simulink model "pid_tune"  (R2022a)
settings: Solver=FixedStepAuto  StartTime=0.0  StopTime=42.0  RelTol=1e-3
libraries: mbedblockslib x6, slpidlib x2, slctrlblks x2, hdlsllib x1
settings Model: PacingRate=2  ExtModeTrigDuration=10  Creator=MATLAB  LastModifiedBy=FUGAZI
settings SolverCC: AutoInsertRateTranBlk=on
settings OptimizationCC: EnhancedBackFolding=on  PassReuseOutputArgsAs=Individual arguments  ZeroExternalMemoryAtStartup=off  ZeroInternalMemoryAtStartup=off  MaxStackSize=64  OptimizeBlockOrder=speed  DifferentSizesBufferReuse=on  OptimizationCustomize=off  EfficientTunableParamExpr=on
settings DebuggingCC: ParameterTunabilityLossMsg=error
settings HardwareCC: ProdBitPerPointer=32  ProdBitPerSizeT=32  ProdBitPerPtrDiffT=32  ProdLargestAtomicInteger=Long  ProdLargestAtomicFloat=Double  ProdWordSize=32  ProdLongLongMode=on  ProdHWDeviceType=ARM Compatible->ARM Cortex
settings SFSimCC: MATLABDynamicMemAlloc=off
settings RTWCC: SystemTargetFile=ert.tlc  HardwareBoard=STM32 Nucleo L476RG  TemplateMakefile=ert_default_tmf  Toolchain=GNU Tools for ARM Embedded Processors
settings CodeAppCC: ForceParamTrailComments=on  IgnoreCustomStorageClasses=off  OperatorAnnotations=on  SimulinkDataObjDesc=on  SFDataObjDesc=on  InsertBlockDesc=on
settings ERTTargetCC: ExtModeTransport=3  ExtModeStaticAlloc=on  ExtModeStaticAllocSize=2000  ExtModeMexFile=ext_xcp  ExtModeIntrfLevel=Level2 - Open

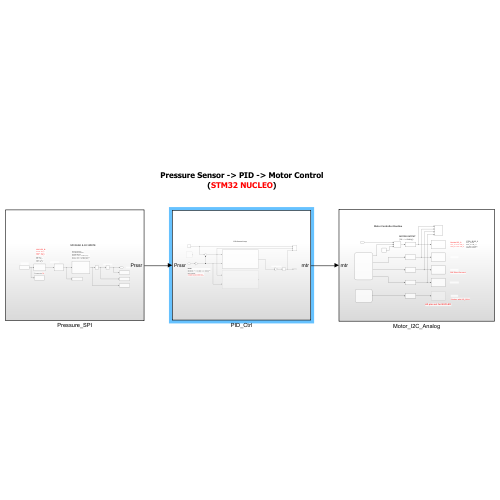
[thumbnail: Simulink's stored preview of the top-level diagram]
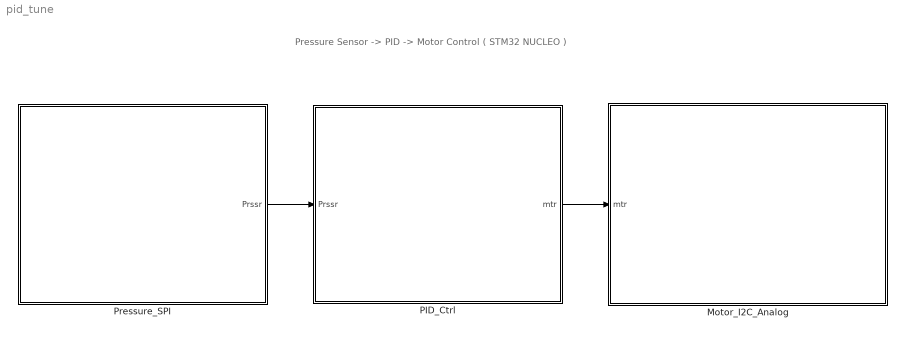
== system pid_tune ==
  note: Pressure Sensor -> PID -> Motor Control
      | ( STM32 NUCLEO )
  Motor_I2C_Analog : Subsystem
  PID_Ctrl : Subsystem
  Pressure_SPI : Subsystem
  wires:
  PID_Ctrl/1(mtr) -> Motor_I2C_Analog/1(mtr)
  Pressure_SPI/1(Prssr) -> PID_Ctrl/1(Prssr)

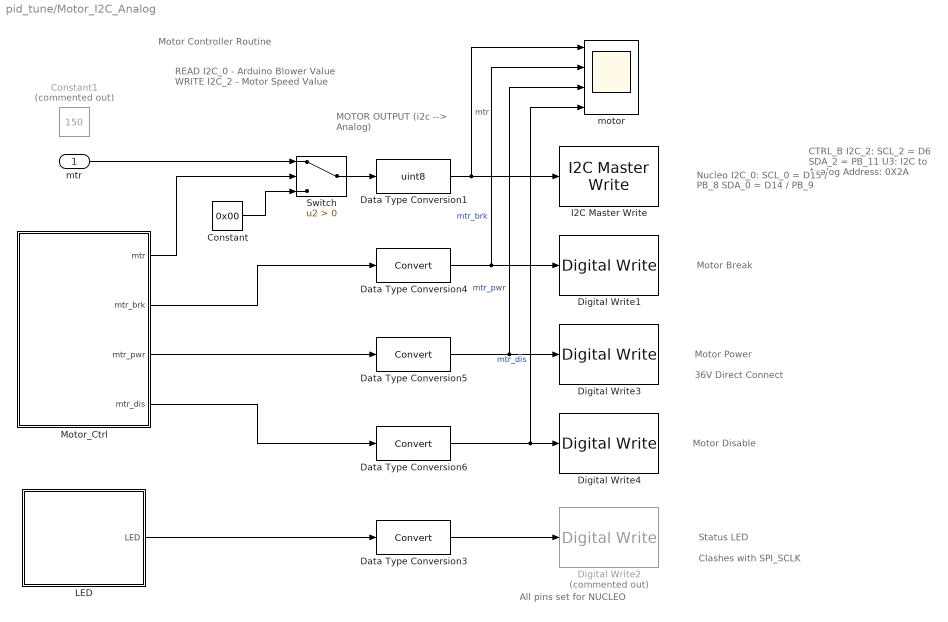
== system pid_tune/Motor_I2C_Analog ==
  note: All pins set for NUCLEO
  note: Motor Controller Routine
  note: Status LED
  note: READ  I2C_0  - Arduino Blower Value
      | WRITE I2C_2 - Motor Speed Value
  note: Motor Power
  note: MOTOR OUTPUT
      | (i2c --> Analog)
  note: Motor Break
  note: Motor Disable
  note: CTRL_B I2C_2:
      | SCL_2 = D6
      | SDA_2 = PB_11
      | U3: I2C to Analog
      | Address: 0X2A
  note: 36V Direct Connect
  note: Nucleo I2C_0:
      | SCL_0 = D15 / PB_8
      | SDA_0 = D14 / PB_9
  note: Clashes with SPI_SCLK
  mtr : Inport
  Constant : Constant  Value=0x00
  Constant1 : Constant  Commented=on  Value=150
  Data Type Conversion1 : DataTypeConversion  OutDataTypeStr=uint8  SaturateOnIntegerOverflow=off  RndMeth=Floor
  Data Type Conversion{3..6} (4 alike) : DataTypeConversion  SaturateOnIntegerOverflow=off  RndMeth=Floor
  Digital Write1 : mbedblockslib/Digital Write  Pin=PA_8  Direction=output
      settings: SourceProductBaseCode=MICROBIT,NUCLEO,STMICRODIS
  Digital Write2 : mbedblockslib/Digital Write  Commented=on  Pin=PA_5  Direction=output
      settings: SourceProductBaseCode=MICROBIT,NUCLEO,STMICRODIS
  Digital Write3 : mbedblockslib/Digital Write  Pin=PB_4  Direction=output
      settings: SourceProductBaseCode=MICROBIT,NUCLEO,STMICRODIS
  Digital Write4 : mbedblockslib/Digital Write  Pin=PB_10  Direction=output
      settings: SourceProductBaseCode=MICROBIT,NUCLEO,STMICRODIS
  I2C Master Write : mbedblockslib/I2C Master Write  I2CModule=0  Mode=Master  SlaveAddress=uint8(hex2dec('2A'))  SlaveByteOrder=BigEndian  Direction=Transmitter  RegisterAddressMode=on  RegisterAddress=uint8(hex2dec('10'))  SlaveDataType=uint8  DataLength=2  NoAck=off  RepeatedStart=off  OutputStatus=off
      settings: SourceProductBaseCode=MICROBIT,NUCLEO,STMICRODIS
  LED : Stateflow chart  TreatAsAtomicUnit=on
  Motor_Ctrl : Stateflow chart  TreatAsAtomicUnit=on
  Switch : Switch  Criteria=u2 > Threshold  SaturateOnIntegerOverflow=off  InputSameDT=off
  motor : Scope  NumInputPorts=4
  wires:
  Data Type Conversion5/1 -> Digital Write3/1, motor/3  "mtr_pwr"
  Switch/1 -> Data Type Conversion1/1
  Motor_Ctrl/1(mtr) -> Switch/2
  Motor_Ctrl/3(mtr_pwr) -> Data Type Conversion5/1
  Data Type Conversion6/1 -> motor/4, Digital Write4/1  "mtr_dis"
  Motor_Ctrl/2(mtr_brk) -> Data Type Conversion4/1
  Data Type Conversion3/1 -> Digital Write2/1
  Motor_Ctrl/4(mtr_dis) -> Data Type Conversion6/1
  Data Type Conversion4/1 -> Digital Write1/1, motor/2  "mtr_brk"
  Data Type Conversion1/1 -> motor/1, I2C Master Write/1  "mtr"
  LED/1(LED) -> Data Type Conversion3/1
  Constant/1 -> Switch/3
  mtr/1 -> Switch/1

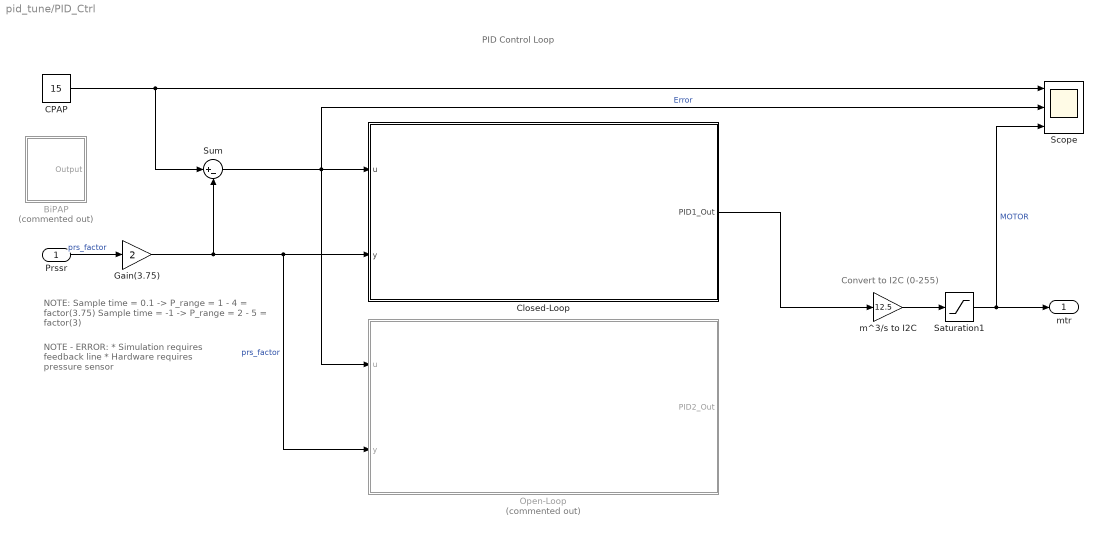
== system pid_tune/PID_Ctrl ==
  note: NOTE:
      | Sample time = 0.1 -> P_range = 1 - 4 = factor(3.75)
      | Sample time = -1 -> P_range = 2 - 5 = factor(3)
  note: PID Control Loop
  note: Convert to I2C (0-255)
  note: NOTE - ERROR:
      | * Simulation requires feedback line
      | * Hardware requires pressure sensor
  Prssr : Inport
  BiPAP : Stateflow chart  Commented=on  TreatAsAtomicUnit=on
  CPAP : Constant  Value=15
  Closed-Loop : Subsystem
  Gain(3.75) : Gain  Gain=2
  Open-Loop : Subsystem  Commented=on
  Saturation1 : Saturate  UpperLimit=180  LowerLimit=0
  Scope : Scope  NumInputPorts=3
  Sum : Sum  Inputs=|+-
  m^3/s to I2C : Gain  Gain=12.5
  mtr : Outport
  wires:
  Saturation1/1 -> Scope/3, mtr/1  "MOTOR"
  m^3/s to I2C/1 -> Saturation1/1
  Prssr/1 -> Gain(3.75)/1  "prs_factor"
  Sum/1 -> Scope/2, Open-Loop/1(u), Closed-Loop/1(u)  "Error"
  Closed-Loop/1(PID1_Out) -> m^3/s to I2C/1
  CPAP/1 -> Sum/1, Scope/1
  Gain(3.75)/1 -> Open-Loop/2(y), Closed-Loop/2(y), Sum/2  "prs_factor"

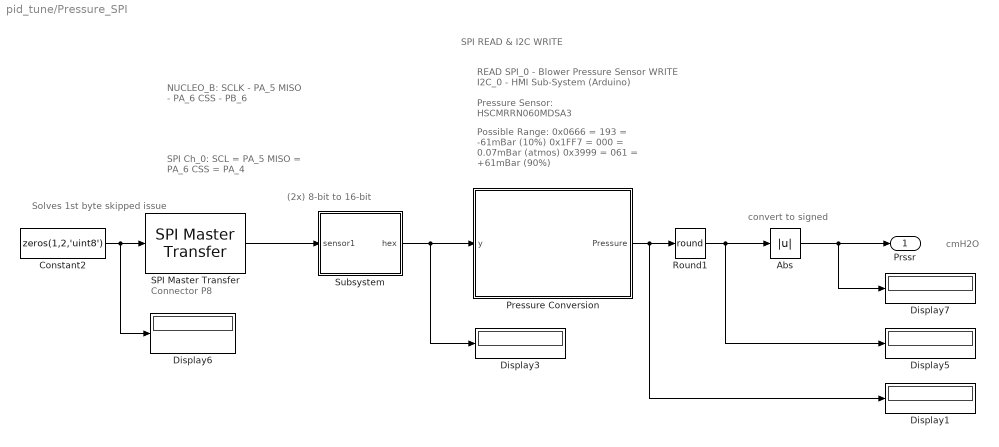
== system pid_tune/Pressure_SPI ==
  note: Pressure Sensor:
      | HSCMRRN060MDSA3
  note: Connector P8
  note: cmH2O
  note: convert to signed
  note: (2x) 8-bit to 16-bit
  note: SPI READ & I2C WRITE
  note: READ SPI_0  -  Blower Pressure Sensor
      | WRITE I2C_0 - HMI Sub-System (Arduino)
  note: SPI Ch_0:
      | SCL = PA_5
      | MISO = PA_6
      | CSS = PA_4
  note: Solves 1st byte
      | skipped issue
  note: Possible Range:
      | 0x0666 = 193 = -61mBar (10%)
      | 0x1FF7 = 000 = 0.07mBar (atmos)
      | 0x3999 = 061 = +61mBar (90%)
  note: NUCLEO_B:
      | SCLK - PA_5
      | MISO - PA_6
      | CSS - PB_6
  Abs : Abs  SaturateOnIntegerOverflow=off
  Constant2 : Constant  Value=zeros(1,2,'uint8')  OutDataTypeStr=uint8  SampleTime=0.1
  Display{1,3,5..7} (5 alike) : Display
      Display3 settings: Format=hex (Stored Integer)
      Display6 settings: Format=hex (Stored Integer)
  Pressure Conversion : Subsystem
  Round1 : Rounding  Operator=round
  SPI Master Transfer : mbedblockslib/SPI Master Transfer  SPIModule=0  Mode=Master  BusSpeed=uint32( 1000000 )  Pin=PB_6  FirstBitToTransfer=Most significant bit (MSB)  ClockMode=0  BlockFunction=Transfer  RegisterAddress=0  OutputDataType=int8  OutputDataLength=1  UseCustomSSPin=Explicit GPIO calls  ActiveLowSSPin=Active low
      settings: SourceProductBaseCode=MICROBIT,NUCLEO,STMICRODIS
  Subsystem : Subsystem
  Prssr : Outport
  wires:
  SPI Master Transfer/1 -> Subsystem/1(sensor1)
  Subsystem/1(hex) -> Pressure Conversion/1(y), Display3/1
  Constant2/1 -> SPI Master Transfer/1, Display6/1
  Round1/1 -> Abs/1, Display5/1
  Pressure Conversion/1(Pressure) -> Display1/1, Round1/1
  Abs/1 -> Display7/1, Prssr/1

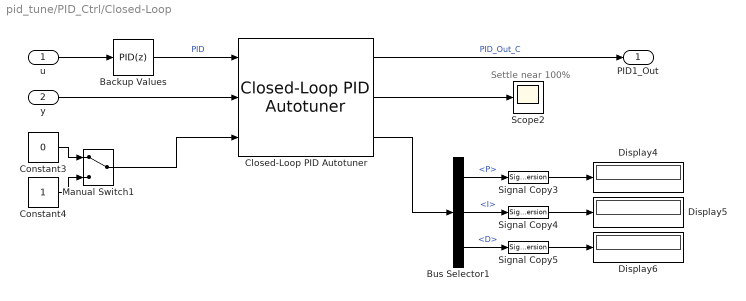
== system pid_tune/PID_Ctrl/Closed-Loop ==
  note: Settle near 100%
  u : Inport
  y : Inport  Port=2
  Backup Values : slpidlib/PID Controller  Controller=PID  Form=Parallel  TimeDomain=Discrete-time  UseExternalTs=off  SampleTime=-1  IntegratorMethod=Forward Euler  FilterMethod=Forward Euler  ControllerParametersSource=internal  P=5  I=25  UseKiTs=off  D=1  N=80  UseFilter=on  TunerSelectOption=Transfer Function Based (PID Tuner App)  InitialConditionSource=internal  InitialConditionForIntegrator=0  InitialConditionForFilter=0  DifferentiatorICPrevScaledInput=0  ExternalReset=none  TrackingMode=off  Kt=1  LimitOutput=off  SatLimitsSource=internal  UpperSaturationLimit=1  LowerSaturationLimit=0  LinearizeAsGain=off  AntiWindupMode=none  Kb=1  POutMin=[]  POutMax=[]  IOutMin=[]  IOutMax=[]  DOutMin=[]  DOutMax=[]  NOutMin=[]  NOutMax=[]  SumOutMin=[]  SumOutMax=[]  SaturationOutMin=[]  SaturationOutMax=[]  PParamMin=[]  PParamMax=[]  IParamMin=[]  IParamMax=[]  DParamMin=[]  DParamMax=[]  NParamMin=[]  NParamMax=[]  KbParamMin=[]  KbParamMax=[]  KtParamMin=[]  KtParamMax=[]  KbOutMin=[]  KbOutMax=[]  KtOutMin=[]  KtOutMax=[]  IntegratorOutMin=[]  IntegratorOutMax=[]  FilterOutMin=[]  FilterOutMax=[]  SumI1OutMin=[]  SumI1OutMax=[]  SumI2OutMin=[]  SumI2OutMax=[]  SumI3OutMin=[]  SumI3OutMax=[]  SumI4OutMin=[]  SumI4OutMax=[]  SumDOutMin=[]  SumDOutMax=[]  DifferentiatorOutMin=[]  DifferentiatorOutMax=[]  FilterDiffOutCoefMin=[]  FilterDiffOutCoefMax=[]  ReciprocalOutMin=[]  ReciprocalOutMax=[]  SumDenOutMin=[]  SumDenOutMax=[]  SumNumOutMin=[]  SumNumOutMax=[]  DivideOutMin=[]  DivideOutMax=[]  UdiffTsProdOutMin=[]  UdiffTsProdOutMax=[]  NTsProdOutMin=[]  NTsProdOutMax=[]  UintegralTsProdOutMin=[]  UintegralTsProdOutMax=[]  UngainTsProdOutMin=[]  UngainTsProdOutMax=[]  IntegratorContinuousStateAttributes=''  IntegratorStateMustResolveToSignalObject=off  IntegratorRTWStateStorageClass=Auto  FilterContinuousStateAttributes=''  FilterStateMustResolveToSignalObject=off  FilterRTWStateStorageClass=Auto  ParallelPVariant=InternalParameters  IdealPVariant=Disabled  IVariant=InternalParameters  DVariant=InternalParameters  IntegratorVariant=Discrete  SatVariant=Disabled  AWVariant=Passthrough  PCopyVariant=Disabled  TRVariant=Disabled  FdbkBlocksVariant=Forward  IdealPFdbkVariant=Disabled  SatFdbkVariant=Disabled  DerivativeFilterVariant=ForwardEulerFilter  NVariant=InternalParameters  NCopyVariant=Disabled  FilterICVariant=InternalICsFilter  IntegratorICVariant=InternalICs  ExternalResetVariant=Disabled  TRSumVariant=Passthrough  SumFdbkVariant=Disabled  SumVariant=Sum_PID  TsampFilterVariant=InternalTs  TsampNgainVariant=Passthrough  TsampIntegralVariant=Passthrough  ExternalSaturationOutDataTypeStr=Inherit: Same as second input  aMode=0
  Bus Selector1 : BusSelector  OutputSignals=P,I,D
  Closed-Loop PID Autotuner : slctrlblks/Closed-Loop PID Autotuner  PIDType=PID  PIDForm=Parallel  TimeDomain=discrete-time  DiscreteTs=-1  TuningTs=0.2  UseTuningTs=off  IntegratorFormula=Forward Euler  FilterFormula=Forward Euler  ContinuousTs=0.02  Bandwidth=28  UseExternalWC=off  TargetPM=45  UseExternalPM=off  UseExternalAchievedPM=off  ExperimentMode=Superposition  PlantType=Stable  PlantSign=Positive  AmpSine=10  UseExternalAmpSine=off  UseExternalFRD=off  UseExternalU0=off  UseCompanion=off  NotDeployTuningModule=off  UsePLCCoder=off  OutputMode=control action + perturbation  BlockDataType=double  UseConnectedPID=on  blockpath=[]  tunedP=0  tunedI=0  tunedD=0  tunedN=100  tunedPM=0  EstimationWindowSize=3  UseExternalTuningParams=off  OutputChoice=VariantCandD  SingleMultiRateVariant=SingleSamplingRate  ExperimentModeVariant=VariantSuperimposed  NumEstimationPeriods=4  NumSettlingPeriods=2
      settings: SourceProductBaseCode=SD
  Constant3 : Constant  Value=0
  Constant4 : Constant
  Display4 : Display
  Display5 : Display
  Display6 : Display
  Manual Switch1 : ManualSwitch
  Scope2 : Scope
  Signal Copy3 : SignalConversion  OverrideOpt=off
  Signal Copy4 : SignalConversion  OverrideOpt=off
  Signal Copy5 : SignalConversion  OverrideOpt=off
  PID1_Out : Outport
  wires:
  Signal Copy4/1 -> Display5/1
  Bus Selector1/3 -> Signal Copy5/1  "<D>"
  Closed-Loop PID Autotuner/1 -> PID1_Out/1  "PID_Out_C"
  Constant4/1 -> Manual Switch1/2
  Constant3/1 -> Manual Switch1/1
  Bus Selector1/2 -> Signal Copy4/1  "<I>"
  Signal Copy3/1 -> Display4/1
  Bus Selector1/1 -> Signal Copy3/1  "<P>"
  u/1 -> Backup Values/1
  Signal Copy5/1 -> Display6/1
  Backup Values/1 -> Closed-Loop PID Autotuner/1  "PID"
  Closed-Loop PID Autotuner/3 -> Bus Selector1/1
  Closed-Loop PID Autotuner/2 -> Scope2/1
  y/1 -> Closed-Loop PID Autotuner/2
  Manual Switch1/1 -> Closed-Loop PID Autotuner/3

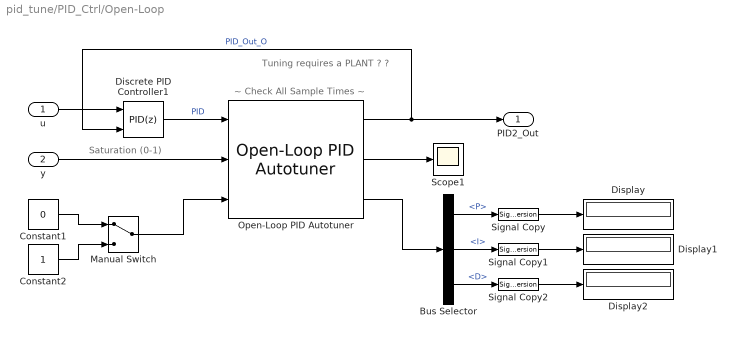
== system pid_tune/PID_Ctrl/Open-Loop ==
  note: Tuning requires
      | a PLANT ? ?
  note: ~ Check All Sample Times ~
  note: Saturation (0-1)
  u : Inport
  y : Inport  Port=2
  Bus Selector : BusSelector  OutputSignals=P,I,D
  Constant1 : Constant  Value=0
  Constant2 : Constant
  Discrete PID Controller1 : slpidlib/PID Controller  Controller=PID  Form=Parallel  TimeDomain=Discrete-time  UseExternalTs=off  SampleTime=-1  IntegratorMethod=Forward Euler  FilterMethod=Forward Euler  ControllerParametersSource=internal  P=90  I=140  UseKiTs=off  D=4  N=100  UseFilter=on  TunerSelectOption=Transfer Function Based (PID Tuner App)  InitialConditionSource=internal  InitialConditionForIntegrator=0  InitialConditionForFilter=0  DifferentiatorICPrevScaledInput=0  ExternalReset=none  TrackingMode=on  Kt=1  LimitOutput=off  SatLimitsSource=internal  UpperSaturationLimit=1  LowerSaturationLimit=0  LinearizeAsGain=off  AntiWindupMode=none  Kb=1  POutMin=[]  POutMax=[]  IOutMin=[]  IOutMax=[]  DOutMin=[]  DOutMax=[]  NOutMin=[]  NOutMax=[]  SumOutMin=[]  SumOutMax=[]  SaturationOutMin=[]  SaturationOutMax=[]  PParamMin=[]  PParamMax=[]  IParamMin=[]  IParamMax=[]  DParamMin=[]  DParamMax=[]  NParamMin=[]  NParamMax=[]  KbParamMin=[]  KbParamMax=[]  KtParamMin=[]  KtParamMax=[]  KbOutMin=[]  KbOutMax=[]  KtOutMin=[]  KtOutMax=[]  IntegratorOutMin=[]  IntegratorOutMax=[]  FilterOutMin=[]  FilterOutMax=[]  SumI1OutMin=[]  SumI1OutMax=[]  SumI2OutMin=[]  SumI2OutMax=[]  SumI3OutMin=[]  SumI3OutMax=[]  SumI4OutMin=[]  SumI4OutMax=[]  SumDOutMin=[]  SumDOutMax=[]  DifferentiatorOutMin=[]  DifferentiatorOutMax=[]  FilterDiffOutCoefMin=[]  FilterDiffOutCoefMax=[]  ReciprocalOutMin=[]  ReciprocalOutMax=[]  SumDenOutMin=[]  SumDenOutMax=[]  SumNumOutMin=[]  SumNumOutMax=[]  DivideOutMin=[]  DivideOutMax=[]  UdiffTsProdOutMin=[]  UdiffTsProdOutMax=[]  NTsProdOutMin=[]  NTsProdOutMax=[]  UintegralTsProdOutMin=[]  UintegralTsProdOutMax=[]  UngainTsProdOutMin=[]  UngainTsProdOutMax=[]  IntegratorContinuousStateAttributes=''  IntegratorStateMustResolveToSignalObject=off  IntegratorRTWStateStorageClass=Auto  FilterContinuousStateAttributes=''  FilterStateMustResolveToSignalObject=off  FilterRTWStateStorageClass=Auto  ParallelPVariant=InternalParameters  IdealPVariant=Disabled  IVariant=InternalParameters  DVariant=InternalParameters  IntegratorVariant=Discrete  SatVariant=Disabled  AWVariant=Passthrough  PCopyVariant=Disabled  TRVariant=Enabled  FdbkBlocksVariant=Forward  IdealPFdbkVariant=Disabled  SatFdbkVariant=Disabled  DerivativeFilterVariant=ForwardEulerFilter  NVariant=InternalParameters  NCopyVariant=Disabled  FilterICVariant=InternalICsFilter  IntegratorICVariant=InternalICs  ExternalResetVariant=Disabled  TRSumVariant=TrackingMode  SumFdbkVariant=Disabled  SumVariant=Sum_PID  TsampFilterVariant=InternalTs  TsampNgainVariant=Passthrough  TsampIntegralVariant=Passthrough  ExternalSaturationOutDataTypeStr=Inherit: Same as second input  aMode=0
  Display : Display
  Display1 : Display
  Display2 : Display
  Manual Switch : ManualSwitch
  Open-Loop PID Autotuner : slctrlblks/Open-Loop PID Autotuner  PIDType=PI  PIDForm=Parallel  TimeDomain=discrete-time  DiscreteTs=0.1  IntegratorFormula=Forward Euler  FilterFormula=Forward Euler  ContinuousTs=0.02  Bandwidth=1  UseExternalWC=off  TargetPM=60  UseExternalPM=off  UseExternalAchievedPM=off  AmpSine=1  UseExternalAmpSine=off  EstimateDCGain=on  AmpStep=1  UseExternalAmpStep=off  UseExternalFRD=off  UseExternalU0=off  UseExternalDCGain=off  NotDeployTuningModule=off  UsePLCCoder=off  BlockDataType=double  UseConnectedPID=on  blockpath=[]  tunedP=0  tunedI=0  tunedD=0  tunedN=100  tunedPM=0  EstimationWindowSize=3
      settings: SourceProductBaseCode=SD
  Scope1 : Scope
  Signal Copy : SignalConversion  OverrideOpt=off
  Signal Copy1 : SignalConversion  OverrideOpt=off
  Signal Copy2 : SignalConversion  OverrideOpt=off
  PID2_Out : Outport
  wires:
  Bus Selector/2 -> Signal Copy1/1  "<I>"
  Bus Selector/1 -> Signal Copy/1  "<P>"
  Constant2/1 -> Manual Switch/2
  Signal Copy/1 -> Display/1
  Open-Loop PID Autotuner/1 -> Discrete PID Controller1/2, PID2_Out/1  "PID_Out_O"
  Signal Copy2/1 -> Display2/1
  Constant1/1 -> Manual Switch/1
  Bus Selector/3 -> Signal Copy2/1  "<D>"
  Signal Copy1/1 -> Display1/1
  Open-Loop PID Autotuner/2 -> Scope1/1
  Discrete PID Controller1/1 -> Open-Loop PID Autotuner/1  "PID"
  Manual Switch/1 -> Open-Loop PID Autotuner/3
  Open-Loop PID Autotuner/3 -> Bus Selector/1
  y/1 -> Open-Loop PID Autotuner/2
  u/1 -> Discrete PID Controller1/1

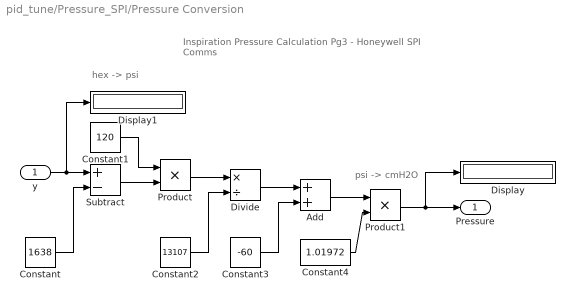
== system pid_tune/Pressure_SPI/Pressure Conversion ==
  note: psi -> cmH2O
  note: Inspiration Pressure Calculation
      | Pg3 - Honeywell SPI Comms
  note: hex -> psi
  y : Inport
  Add : Sum
  Constant : Constant  Value=1638
  Constant1 : Constant  Value=120
  Constant2 : Constant  Value=13107
  Constant3 : Constant  Value=-60
  Constant4 : Constant  Value=1.01972
  Display : Display
  Display1 : Display
      settings: Format=hex (Stored Integer)
  Divide : Product  Inputs=*/
  Product : Product
  Product1 : Product
  Subtract : Sum  Inputs=+-
  Pressure : Outport
  wires:
  Constant/1 -> Subtract/2
  Subtract/1 -> Product/2
  Constant1/1 -> Product/1
  Product/1 -> Divide/1
  Constant2/1 -> Divide/2
  Constant3/1 -> Add/2
  Divide/1 -> Add/1
  Add/1 -> Product1/1
  Constant4/1 -> Product1/2
  Product1/1 -> Pressure/1, Display/1
  y/1 -> Display1/1, Subtract/1

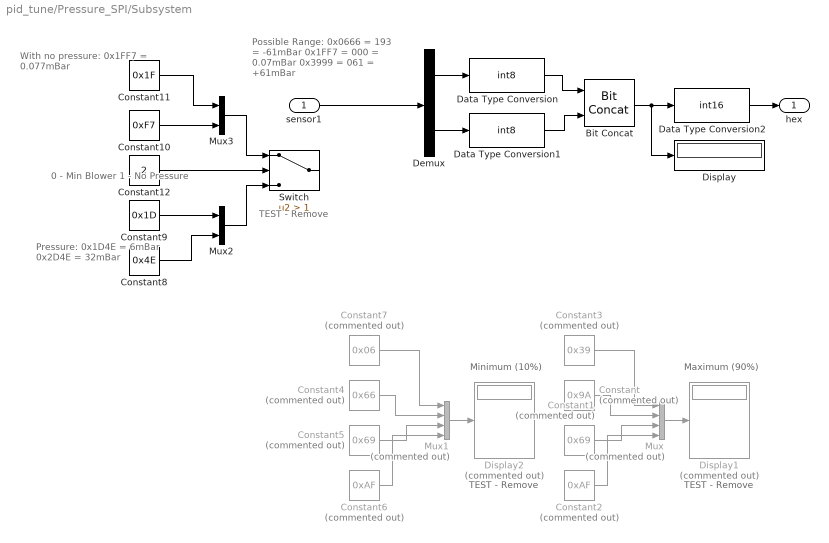
== system pid_tune/Pressure_SPI/Subsystem ==
  note: TEST - Remove
  note: 0 - Min Blower
      | 1 - No Pressure
  note: With no pressure:
      | 0x1FF7 = 0.077mBar
  note: Maximum (90%)
  note: Minimum (10%)
  note: Possible Range:
      | 0x0666 = 193 = -61mBar
      | 0x1FF7 = 000 = 0.07mBar
      | 0x3999 = 061 = +61mBar
  note: Pressure:
      | 0x1D4E = 6mBar
      | 0x2D4E = 32mBar
  note: TEST - Remove
  note: TEST - Remove
  sensor1 : Inport
  Bit Concat : hdlsllib/Logic and Bit Operations/Bit Concat  numInputs=2
  Constant : Constant  Commented=on  Value=0x9A
  Constant1 : Constant  Commented=on  Value=0x69
  Constant10 : Constant  Value=0xF7
  Constant11 : Constant  Value=0x1F
  Constant12 : Constant  Value=2
  Constant2 : Constant  Commented=on  Value=0xAF
  Constant3 : Constant  Commented=on  Value=0x39
  Constant4 : Constant  Commented=on  Value=0x66
  Constant5 : Constant  Commented=on  Value=0x69
  Constant6 : Constant  Commented=on  Value=0xAF
  Constant7 : Constant  Commented=on  Value=0x06
  Constant8 : Constant  Value=0x4E
  Constant9 : Constant  Value=0x1D
  Data Type Conversion : DataTypeConversion  OutDataTypeStr=int8  SaturateOnIntegerOverflow=off  RndMeth=Floor
  Data Type Conversion1 : DataTypeConversion  OutDataTypeStr=int8  SaturateOnIntegerOverflow=off  RndMeth=Floor
  Data Type Conversion2 : DataTypeConversion  OutDataTypeStr=int16  SaturateOnIntegerOverflow=off  RndMeth=Floor
  Demux : Demux  Outputs=2
  Display : Display
      settings: Format=hex (Stored Integer)
  Display1 : Display  Commented=on
      settings: Format=hex (Stored Integer)
  Display2 : Display  Commented=on
      settings: Format=hex (Stored Integer)
  Mux : Mux  Commented=on
  Mux1 : Mux  Commented=on
  Mux2 : Mux  Inputs=2
  Mux3 : Mux  Inputs=2
  Switch : Switch  Criteria=u2 > Threshold  Threshold=1  SaturateOnIntegerOverflow=off  InputSameDT=off
  hex : Outport
  wires:
  Constant3/1 -> Mux/1
  Constant/1 -> Mux/2
  Constant1/1 -> Mux/3
  Constant2/1 -> Mux/4
  Data Type Conversion/1 -> Bit Concat/1
  Data Type Conversion1/1 -> Bit Concat/2
  Demux/1 -> Data Type Conversion/1
  Demux/2 -> Data Type Conversion1/1
  Bit Concat/1 -> Display/1, Data Type Conversion2/1
  Mux/1 -> Display1/1
  Mux1/1 -> Display2/1
  Constant7/1 -> Mux1/1
  Constant6/1 -> Mux1/4
  Constant5/1 -> Mux1/3
  Constant4/1 -> Mux1/2
  Constant9/1 -> Mux2/1
  Constant8/1 -> Mux2/2
  Constant10/1 -> Mux3/2
  Constant11/1 -> Mux3/1
  Constant12/1 -> Switch/2
  Mux3/1 -> Switch/1
  Mux2/1 -> Switch/3
  Data Type Conversion2/1 -> hex/1
  sensor1/1 -> Demux/1

== stateflow chart pid_tune/Motor_I2C_Analog/Motor_Ctrl ==
  state STARTUP % Blower Start
    state Start_1 % Main Power
      entry:
      mtr_pwr = 1; % ON
      exit:
    state Start_2 % Motor Brake
      entry:
      mtr_brk = 1; % Disable
      mtr_dis = 1; % Enabled
      exit:
    (default) -> Start_1 % Main Power
    Start_1 % Main Power -> Start_2 % Motor Brake : after(1,sec)
  state Run_Mtr %
    entry: mtr =1;
    exit:
  note: Shut-Down:
      | after(120,sec)
  state SHUTDOWN % Blower Off
    state Stop_1 % I2C to Anal.
      entry: mtr = 0;
      exit:
    state Stop_2 % Motor Brake
      entry:
      mtr_brk = 0; % Enable
      exit:
    state Stop_3 % Motor Disable
      entry:
      mtr_dis = 0; % Disable
      exit:
    state Stop_4 % Main Power
      entry:
      mtr_pwr = 0; % OFF
      exit:
    (default) -> Stop_1 % I2C to Anal.
    Stop_1 % I2C to Anal. -> Stop_2 % Motor Brake : after(500,msec)
    Stop_2 % Motor Brake -> Stop_3 % Motor Disable : after(500,msec)
    Stop_3 % Motor Disable -> Stop_4 % Main Power : after(500,msec)
  note: 1. Power - On
      | 2. Brake - Off
      | 3. Disable - Off
      | 4. Voltage Output
  note: BRAKE PIN:
      | Enabled = <0.8V or Gnd
      | Deactivated = >2.4V or Not wired
  note: DISABLE PIN:
      | Disable = <0.8V or Gnd
      | Enable = >2.4V or Not wired
  (default) -> STARTUP % Blower Start
  STARTUP % Blower Start -> Run_Mtr % : after(2,sec)
  Run_Mtr % -> SHUTDOWN % Blower Off : after(36,sec)
  data: mtr output; mtr_brk output; mtr_pwr output; mtr_dis output

== stateflow chart pid_tune/Motor_I2C_Analog/LED ==
  state Run % Parent
    state Check % Check Sub-Systems
      entry:
      LED = 0; % LED Off
      exit:
    state LED % Child
      entry: % none
      LED = 1; % LED On
      exit: % none
    (default) -> LED % Child
    LED % Child -> Check % Check Sub-Systems : after(2,sec)
    Check % Check Sub-Systems -> LED % Child : after(2,sec)
  note: Check Input
      | Power present?
  note: TEST:
      | Routine Checks
  (default) -> Run % Parent
  data: LED output

== stateflow chart pid_tune/PID_Ctrl/BiPAP ==
  note: Pressure(6)
      | IPAP(22)  = mtr(200)
      | EPAP(14) = mtr(100)
  state IPAP_out
    entry:
    during:
    Output = 15;%=IPAP;
    exit:
  note: Inhale:
      | IPAP(15)
      | after(2.6,sec)
  note: Exhale:
      | EPAP(5)
      | after(1.4,sec)
  state EPAP_out
    entry:
    during:
    Output = 5;%=EPAP;
    exit:
  (default) -> IPAP_out
  EPAP_out -> IPAP_out : after(3.6,sec)
  IPAP_out -> EPAP_out : after(2.4,sec)
  data: Output output
